simulink model "BMS"  (R2024a)
settings: Solver=VariableStepDiscrete  StartTime=0.0  StopTime=10.0  RelTol=1e-3
undefined symbols (not defined in the file): C1, R0, R1, Ts
settings Model: Creator=pc  LastModifiedBy=pc

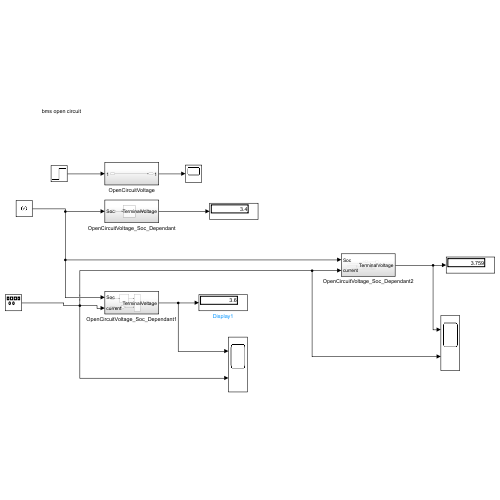
[thumbnail: Simulink's stored preview of the top-level diagram]
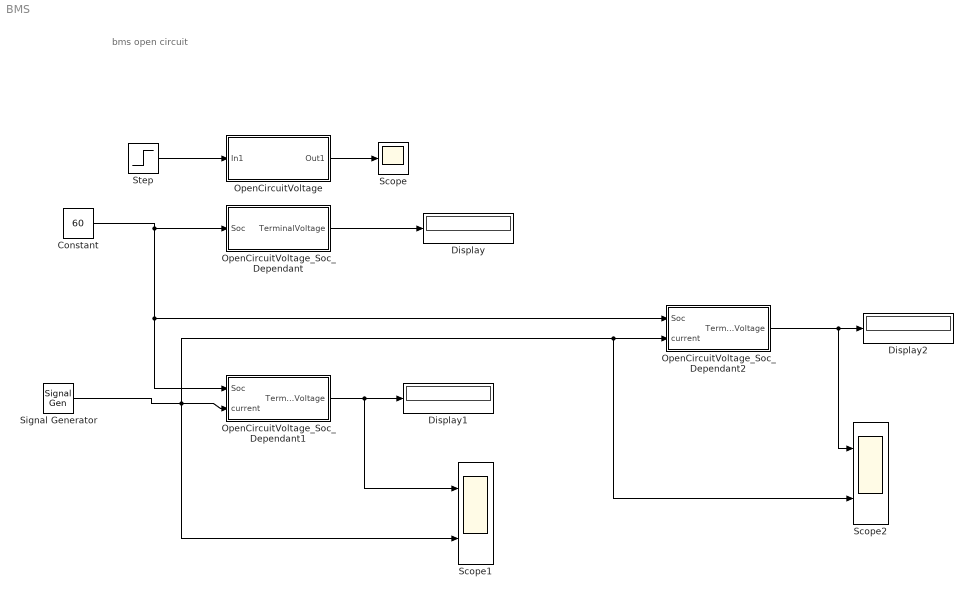
== system BMS ==
  note: bms open circuit
  Constant : Constant  Value=60
  Display : Display
  Display1 : Display
  Display2 : Display
  OpenCircuitVoltage : Subsystem
  OpenCircuitVoltage_Soc_Dependant : Subsystem
  OpenCircuitVoltage_Soc_Dependant1 : Subsystem
  OpenCircuitVoltage_Soc_Dependant2 : Subsystem
  Scope : Scope
  Scope1 : Scope  NumInputPorts=2
  Scope2 : Scope  NumInputPorts=2
  Signal Generator : SignalGenerator  WaveForm=square  Amplitude=20  Frequency=2  Units=rad/sec
  Step : Step  Time=0  Before=2.7  After=2.7  SampleTime=0
  wires:
  Step/1 -> OpenCircuitVoltage/1(In1)
  OpenCircuitVoltage/1(Out1) -> Scope/1
  OpenCircuitVoltage_Soc_Dependant/1(TerminalVoltage) -> Display/1
  Constant/1 -> OpenCircuitVoltage_Soc_Dependant2/1(Soc), OpenCircuitVoltage_Soc_Dependant1/1(Soc), OpenCircuitVoltage_Soc_Dependant/1(Soc)
  OpenCircuitVoltage_Soc_Dependant1/1(TerminalVoltage) -> Scope1/1, Display1/1
  Signal Generator/1 -> OpenCircuitVoltage_Soc_Dependant2/2(current), Scope2/2, Scope1/2, OpenCircuitVoltage_Soc_Dependant1/2(current)
  OpenCircuitVoltage_Soc_Dependant2/1(TerminalVoltage) -> Scope2/1, Display2/1

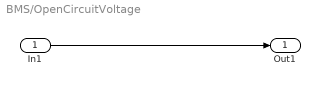
== system BMS/OpenCircuitVoltage ==
  In1 : Inport
  Out1 : Outport
  wires:
  In1/1 -> Out1/1

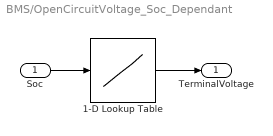
== system BMS/OpenCircuitVoltage_Soc_Dependant ==
  Soc : Inport
  1-D Lookup Table : Lookup_n-D  NumberOfTableDimensions=1  BreakpointsForDimension1=[40,50,60,70,80,100]  Table=[3,3.1,3.4,3.7 ,4,4.2]  InternalRulePriority=Speed  RndMeth=Simplest
  TerminalVoltage : Outport
  wires:
  Soc/1 -> 1-D Lookup Table/1
  1-D Lookup Table/1 -> TerminalVoltage/1

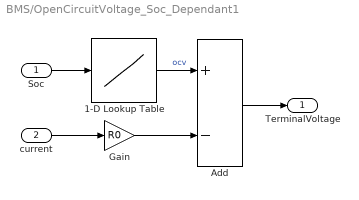
== system BMS/OpenCircuitVoltage_Soc_Dependant1 ==
  Soc : Inport
  current : Inport  Port=2
  1-D Lookup Table : Lookup_n-D  NumberOfTableDimensions=1  BreakpointsForDimension1=[40,50,60,70,80,100]  Table=[3,3.1,3.4,3.7 ,4,4.2]  InternalRulePriority=Speed  RndMeth=Simplest
  Add : Sum  Inputs=+-
  Gain : Gain  Gain=R0
  TerminalVoltage : Outport
  wires:
  Gain/1 -> Add/2
  current/1 -> Gain/1
  Soc/1 -> 1-D Lookup Table/1
  1-D Lookup Table/1 -> Add/1  "ocv"
  Add/1 -> TerminalVoltage/1

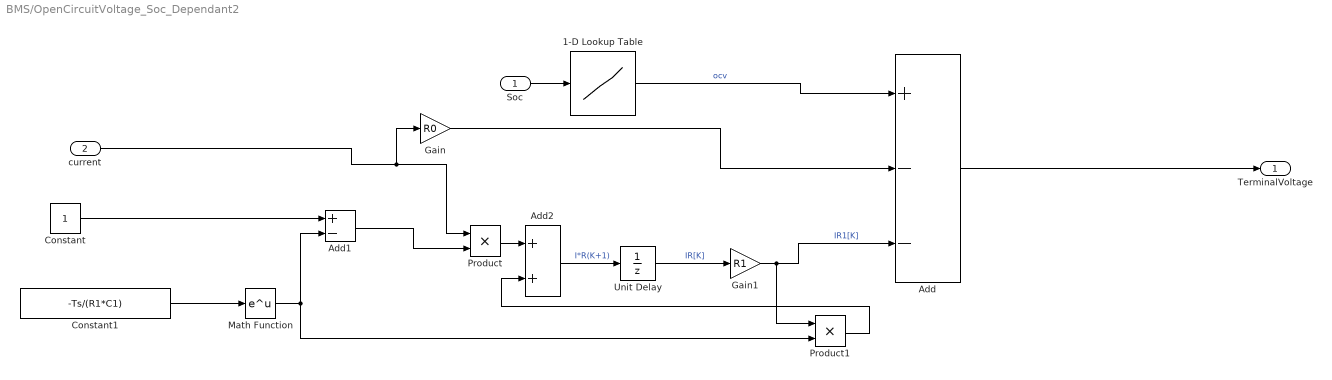
== system BMS/OpenCircuitVoltage_Soc_Dependant2 ==
  Soc : Inport
  current : Inport  Port=2
  1-D Lookup Table : Lookup_n-D  NumberOfTableDimensions=1  BreakpointsForDimension1=[40,50,60,70,80,100]  Table=[3,3.1,3.4,3.7 ,4,4.2]  InternalRulePriority=Speed  RndMeth=Simplest
  Add : Sum  Inputs=+--
  Add1 : Sum  Inputs=+-
  Add2 : Sum
  Constant : Constant
  Constant1 : Constant  Value=-Ts/(R1*C1)
  Gain : Gain  Gain=R0
  Gain1 : Gain  Gain=R1
  Math Function : Math
  Product : Product
  Product1 : Product
  Unit Delay : UnitDelay  SampleTime=-1  HasFrameUpgradeWarning=on
  TerminalVoltage : Outport
  wires:
  Add/1 -> TerminalVoltage/1
  1-D Lookup Table/1 -> Add/1  "ocv"
  Soc/1 -> 1-D Lookup Table/1
  current/1 -> Product/1, Gain/1
  Gain/1 -> Add/2
  Constant/1 -> Add1/1
  Constant1/1 -> Math Function/1
  Math Function/1 -> Add1/2, Product1/2
  Add1/1 -> Product/2
  Product/1 -> Add2/1
  Add2/1 -> Unit Delay/1  "I*R(K+1)"
  Unit Delay/1 -> Gain1/1  "IR[K]"
  Gain1/1 -> Product1/1, Add/3  "IR1[K]"
  Product1/1 -> Add2/2
